simulink model "ECCE_demo1_model"  (R2020a)
settings: Solver=ode23t  StartTime=0.0  StopTime=10/60  MaxStep=50e-6  RelTol=1e-3  AbsTol=1e-3  EnableMultiTasking=on
libraries: powerlib x17
settings Model: Creator=Raymundo  LastModifiedBy=Renata
settings SolverCC: AutoScaleAbsTol=off  MaxConsecutiveMinStep=50  ZeroCrossAlgorithm=Adaptive
settings DataIOCC: ReturnWorkspaceOutputs=off
settings OptimizationCC: LifeSpan=inf
settings DebuggingCC: SFUnexpectedBacktrackingDiag=warning  SFNoUnconditionalDefaultTransitionDiag=warning  ArithmeticOperatorsInVariantConditions=warning
settings SFSimCC: SimUseLocalCustomCode=off  CustomCodeUndefinedFunction=UseInterfaceOnly
settings RTWCC: RTWUseLocalCustomCode=off
settings CodeAppCC: StateflowObjectComments=on
settings GRTTargetCC: TargetLangStandard=C89/C90 (ANSI)
settings ConfigComp: CovMetricSettings=dw  CovHtmlReporting=on  CovSaveCumulativeToWorkspaceVar=on  CovSaveSingleToWorkspaceVar=on  CovExternalEMLEnable=off
settings SimscapeCC: SimscapeNormalizeSystem=off

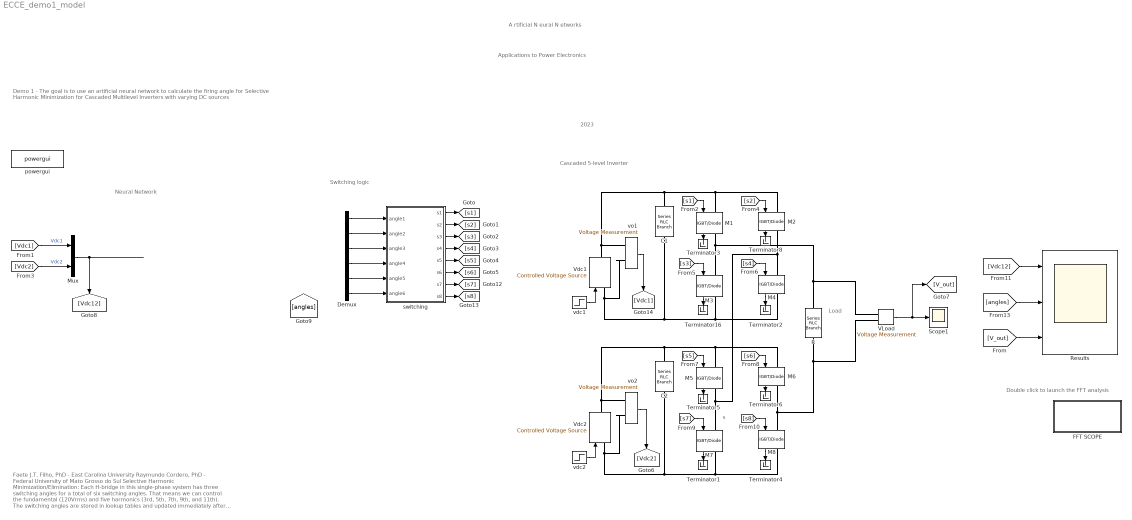
== system ECCE_demo1_model ==
  note: Double click to launch the FFT analysis
  note: Demo 1 - The goal is to use an artificial neural network to calculate the firing angle for Selective Harmonic Minimization for Cascaded Multilevel Inverters with varying DC sources
  note: Switching logic
  note: 2023
  note: A rtificial N eural N etworks
  note: Load
  note: Faete J.T. Filho, PhD - East Carolina University
      | Raymundo Cordero, PhD - Federal University of Mato Grosso do Sul
      |
      | Selective Harmonic Minimization/Elimination: Each H-bridge in this single-phase system has three switching angles for a total of six switching angles. That means we can control the fundamental (120Vrms) and five harmonics (3rd, 5th, 7th, 9th, and 11th). The switching angles are stored in lookup tables and updated immediately after the voltage changes, thus causing some harmonic distortion until a full cycle completes. The range of input voltage for which the harmonics are minimized/eliminated is from 110V to 140V.
      | Range of acceptable input voltage (Vdc1 & Vdc2) for SHE algorithm: 110V to 140V
  note: s
  note: Applications to Power Electronics
  note: Neural Network
  note: Cascaded 5-level Inverter
  C1 : powerlib/Elements/Series RLC Branch  LConnTagsString=__new0  RConnTagsString=__new0  BranchType=RC  Resistance=0.0001  Inductance=1e-3  SetiL0=off  InitialCurrent=0  Capacitance=5600e-6  Setx0=off  InitialVoltage=0  Measurements=None
  C2 : powerlib/Elements/Series RLC Branch  LConnTagsString=__new0  RConnTagsString=__new0  BranchType=RC  Resistance=0.0001  Inductance=1e-3  SetiL0=off  InitialCurrent=0  Capacitance=5600e-6  Setx0=off  InitialVoltage=0  Measurements=None
  Demux : Demux  Outputs=6
  FFT SCOPE : Subsystem
      settings: OpenFcn=power_fftscope
  M{1..8} (8 alike) : powerlib/Power Electronics/IGBT//Diode  Ron=1e-3  Rs=1e5  Cs=inf  Measurements=on
  Mux : Mux  Inputs=2
  R : powerlib/Elements/Series RLC Branch  LConnTagsString=__new0  RConnTagsString=__new0  BranchType=R  Resistance=100  Inductance=1e-3  SetiL0=off  InitialCurrent=0  Capacitance=5600e-6  Setx0=off  InitialVoltage=0  Measurements=None
  Results : Scope  NumInputPorts=3
  Scope1 : Scope
  Terminator{1..6,8,16} (8 alike) : Terminator
  VLoad : powerlib/Measurements/Voltage Measurement  PhasorSimulation=off  OutputType=Complex  PSBequivalent=0
  Vdc1 : powerlib/Electrical Sources/Controlled Voltage Source  Initialize=on  Source_Type=AC  Amplitude=0  Phase=0  Frequency=0  Measurements=None
  Vdc2 : powerlib/Electrical Sources/Controlled Voltage Source  Initialize=on  Source_Type=AC  Amplitude=0  Phase=0  Frequency=0  Measurements=None
  powergui : powerlib/powergui  Priority=1  SimulationMode=Continuous  SampleTime=50e-6  frequency=60  Iterations=50  frequencyindice=0  Pbase=100e6  ErrMax=1e-4  UnitsV=kV  UnitsW=MW  buscounter=0  FunctionMessages=off  echomessages=off  EnableUseOfTLC=off  CurrentSourceSwitches=off  DisableSnubberDevices=off  DisableRonSwitches=off  DisableVfSwitches=off  DisplayEquations=off  AutomaticDiscreteSolvers=off  SolverType=Tustin/Backward Euler (TBE)  Interpol=off  ExternalGateDelay=off  methode=off  Ts=100  x0status=blocks  SPID=on  SwTol=0  HookPort=off  NonlinearTolerance=1e-4  nMaxIteration=100  ContinueOnMaxIteration=off  RestoreLinks=warning  ResistiveCurrentMeasurement=off  Frange=[0:2:500]  Ylog=off  Xlog=on  ShowGrid=off  save=off  variable=ZData  structure=V_load  ZoomFFT=off  StartTime=0.1  cycles=3  DisplayStyle=1  fundamental=60  FreqAxis=on  MaxFrequency=2000  frequencyindicesteady=1  RmsSteady=1  display=off
  switching : Subsystem
  vdc1 : Step  Time=0.1  Before=115  After=130  SampleTime=0
  vdc2 : Step  Time=0.1  Before=125  After=135  SampleTime=0
  vo1 : powerlib/Measurements/Voltage Measurement  PhasorSimulation=off  OutputType=Complex  PSBequivalent=0
  vo2 : powerlib/Measurements/Voltage Measurement  PhasorSimulation=off  OutputType=Complex  PSBequivalent=0
  wires:
  M1/1 -> Terminator3/1
  M2/1 -> Terminator8/1
  [s1] -> M1/1
  [s2] -> M2/1
  [s3] -> M3/1
  [s4] -> M4/1
  [Vdc1] -> Mux/1  "Vdc1"
  [Vdc2] -> Mux/2  "Vdc2"
  vdc1/1 -> Vdc1/1
  Mux/1 -> [Vdc12]
  M4/1 -> Terminator2/1
  M3/1 -> Terminator16/1
  vo1/1 -> [Vdc1]
  M5/1 -> Terminator5/1
  M6/1 -> Terminator6/1
  [s5] -> M5/1
  [s6] -> M6/1
  [s7] -> M7/1
  [s8] -> M8/1
  vdc2/1 -> Vdc2/1
  M8/1 -> Terminator4/1
  M7/1 -> Terminator1/1
  vo2/1 -> [Vdc2]
  switching/1(s1) -> [s1]
  switching/2(s2) -> [s2]
  switching/3(s3) -> [s3]
  switching/4(s4) -> [s4]
  switching/5(s5) -> [s5]
  switching/6(s6) -> [s6]
  switching/7(s7) -> [s7]
  switching/8(s8) -> [s8]
  Demux/1 -> switching/1(angle1)
  Demux/2 -> switching/2(angle2)
  Demux/3 -> switching/3(angle3)
  Demux/4 -> switching/4(angle4)
  Demux/5 -> switching/5(angle5)
  Demux/6 -> switching/6(angle6)
  VLoad/1 -> Scope1/1, [V_out]
  ? -> Demux/1, [angles]  "Firing angle"
  [Vdc12] -> Results/1
  [V_out] -> Results/3
  [angles] -> Results/2
  connections:
  M2/LConn1 -- Vdc1/RConn1 -- vo1/LConn1 -- C1/LConn1 -- M1/LConn1
  C1/RConn1 -- Vdc1/LConn1 -- vo1/LConn2 -- M4/RConn1 -- M3/RConn1
  Vdc2/RConn1 -- vo2/LConn1 -- C2/LConn1 -- M5/LConn1 -- M6/LConn1
  Vdc2/LConn1 -- vo2/LConn2 -- C2/RConn1 -- M7/RConn1 -- M8/RConn1
  M1/RConn1 -- VLoad/LConn1 -- R/RConn1 -- M3/LConn1
  M7/LConn1 -- M4/LConn1 -- M2/RConn1 -- M5/RConn1
  M6/RConn1 -- R/LConn1 -- VLoad/LConn2 -- M8/LConn1

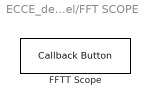
== system ECCE_demo1_model/FFT SCOPE ==
  FFTT Scope : CallbackButton  ButtonText=FFT analysis
      settings: ClickFcn=power_fftscope

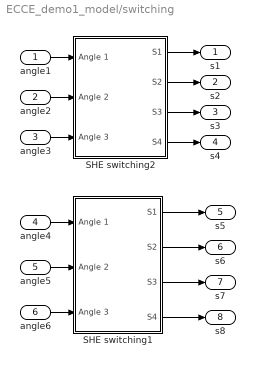
== system ECCE_demo1_model/switching ==
  angle1 : Inport
  angle2 : Inport  Port=2
  angle3 : Inport  Port=3
  angle4 : Inport  Port=4
  angle5 : Inport  Port=5
  angle6 : Inport  Port=6
  SHE switching1 : Subsystem
  SHE switching2 : Subsystem
  s1 : Outport
  s2 : Outport  Port=2
  s3 : Outport  Port=3
  s4 : Outport  Port=4
  s5 : Outport  Port=5
  s6 : Outport  Port=6
  s7 : Outport  Port=7
  s8 : Outport  Port=8
  wires:
  SHE switching2/1(S1) -> s1/1
  SHE switching1/1(S1) -> s5/1
  SHE switching2/4(S4) -> s4/1
  SHE switching1/4(S4) -> s8/1
  SHE switching2/2(S2) -> s2/1
  SHE switching2/3(S3) -> s3/1
  SHE switching1/3(S3) -> s7/1
  SHE switching1/2(S2) -> s6/1
  angle4/1 -> SHE switching1/1(Angle 1)
  angle6/1 -> SHE switching1/3(Angle 3)
  angle2/1 -> SHE switching2/2(Angle 2)
  angle5/1 -> SHE switching1/2(Angle 2)
  angle3/1 -> SHE switching2/3(Angle 3)
  angle1/1 -> SHE switching2/1(Angle 1)

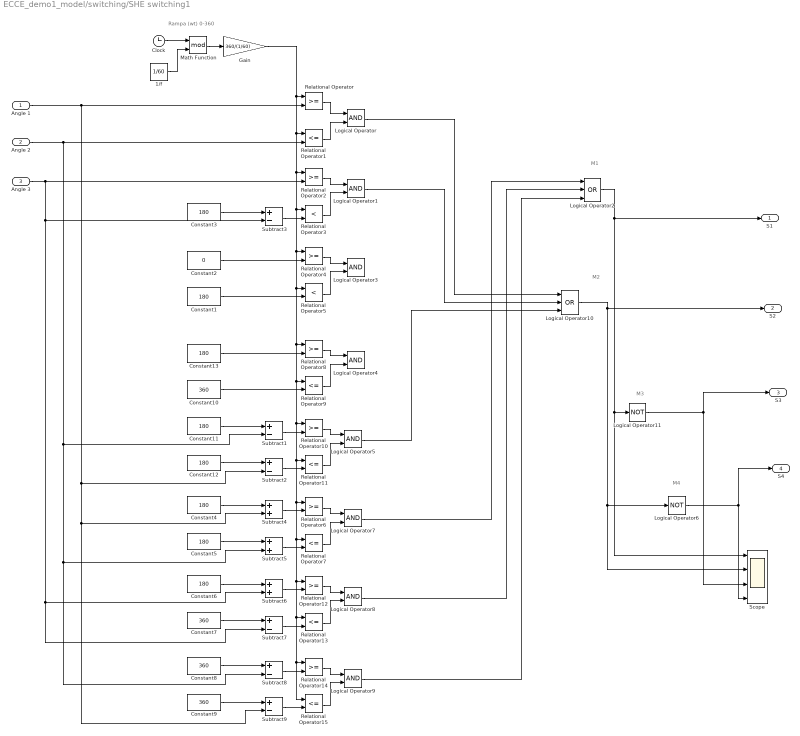
== system ECCE_demo1_model/switching/SHE switching1 ==
  note: M4
  note: M3
  note: M2
  note: M1
  note: Rampa (wt) 0-360
  Angle 1 : Inport
  Angle 2 : Inport  Port=2
  Angle 3 : Inport  Port=3
  1/f : Constant  Value=1/60
  Clock : Clock
  Constant{1,3..6,11..13} (8 alike) : Constant  Value=180
  Constant{7..10} (4 alike) : Constant  Value=360
  Constant2 : Constant  Value=0
  Gain : Gain  Gain=360/(1/60)
  Logical Operator{,1,3..5,7..9} (8 alike) : Logic  AllPortsSameDT=off  OutDataTypeStr=boolean
  Logical Operator10 : Logic  Operator=OR  Inputs=3  AllPortsSameDT=off  OutDataTypeStr=boolean
  Logical Operator11 : Logic  Operator=NOT  AllPortsSameDT=off  OutDataTypeStr=boolean
  Logical Operator2 : Logic  Operator=OR  Inputs=3  AllPortsSameDT=off  OutDataTypeStr=boolean
  Logical Operator6 : Logic  Operator=NOT  AllPortsSameDT=off  OutDataTypeStr=boolean
  Math Function : Math  Operator=mod  SignedPower=on  SaturateOnIntegerOverflow=on
  Relational Operator{,2,4,6,8,10,12,14} (8 alike) : RelationalOperator  OutDataTypeStr=boolean  RndMeth=Nearest
  Relational Operator{1,7,9,11,13,15} (6 alike) : RelationalOperator  Operator=<=  OutDataTypeStr=boolean  RndMeth=Nearest
  Relational Operator3 : RelationalOperator  Operator=<  OutDataTypeStr=boolean  RndMeth=Nearest
  Relational Operator5 : RelationalOperator  Operator=<  OutDataTypeStr=boolean  RndMeth=Nearest
  Scope : Scope  NumInputPorts=4
  Subtract{1..3,7..9} (6 alike) : Sum  Inputs=+-
  Subtract4 : Sum
  Subtract5 : Sum
  Subtract6 : Sum
  S1 : Outport
  S2 : Outport  Port=2
  S3 : Outport  Port=3
  S4 : Outport  Port=4
  wires:
  Gain/1 -> Relational Operator2/1, Relational Operator3/1, Relational Operator4/1, Relational Operator5/1, Relational Operator10/1, Relational Operator15/1, Relational Operator14/1, Relational Operator13/1, Relational Operator12/1, Relational Operator7/1, Relational Operator6/1, Relational Operator11/1, Relational Operator9/1, Relational Operator8/1, Relational Operator1/1, Relational Operator/1
  Relational Operator3/1 -> Logical Operator1/2
  Relational Operator10/1 -> Logical Operator5/1
  Relational Operator8/1 -> Logical Operator4/1
  1/f/1 -> Math Function/2
  Relational Operator1/1 -> Logical Operator/2
  Relational Operator2/1 -> Logical Operator1/1
  Relational Operator/1 -> Logical Operator/1
  Clock/1 -> Math Function/1
  Relational Operator11/1 -> Logical Operator5/2
  Relational Operator9/1 -> Logical Operator4/2
  Math Function/1 -> Gain/1
  Constant11/1 -> Subtract1/1
  Subtract1/1 -> Relational Operator10/2
  Subtract2/1 -> Relational Operator11/2
  Constant12/1 -> Subtract2/1
  Relational Operator4/1 -> Logical Operator3/1
  Relational Operator5/1 -> Logical Operator3/2
  Constant1/1 -> Relational Operator5/2
  Constant2/1 -> Relational Operator4/2
  Constant3/1 -> Subtract3/1
  Subtract3/1 -> Relational Operator3/2
  Constant5/1 -> Subtract5/1
  Subtract5/1 -> Relational Operator7/2
  Subtract4/1 -> Relational Operator6/2
  Constant4/1 -> Subtract4/1
  Relational Operator7/1 -> Logical Operator7/2
  Relational Operator6/1 -> Logical Operator7/1
  Relational Operator12/1 -> Logical Operator8/1
  Relational Operator13/1 -> Logical Operator8/2
  Constant6/1 -> Subtract6/1
  Subtract6/1 -> Relational Operator12/2
  Subtract7/1 -> Relational Operator13/2
  Angle 3/1 -> Relational Operator2/2, Subtract3/2, Subtract7/2, Subtract6/2
  Constant7/1 -> Subtract7/1
  Constant9/1 -> Subtract9/1
  Angle 1/1 -> Subtract9/2, Subtract4/2, Subtract2/2, Relational Operator/2
  Subtract9/1 -> Relational Operator15/2
  Subtract8/1 -> Relational Operator14/2
  Constant8/1 -> Subtract8/1
  Angle 2/1 -> Subtract8/2, Subtract5/2, Subtract1/2, Relational Operator1/2
  Relational Operator15/1 -> Logical Operator9/2
  Relational Operator14/1 -> Logical Operator9/1
  Logical Operator/1 -> Logical Operator10/1
  Logical Operator1/1 -> Logical Operator10/2
  Logical Operator5/1 -> Logical Operator10/3
  Logical Operator7/1 -> Logical Operator2/1
  Logical Operator8/1 -> Logical Operator2/2
  Logical Operator9/1 -> Logical Operator2/3
  Constant13/1 -> Relational Operator8/2
  Constant10/1 -> Relational Operator9/2
  Logical Operator2/1 -> Scope/1, Logical Operator11/1, S1/1
  Logical Operator10/1 -> Scope/2, Logical Operator6/1, S2/1
  Logical Operator11/1 -> S3/1, Scope/3
  Logical Operator6/1 -> Scope/4, S4/1

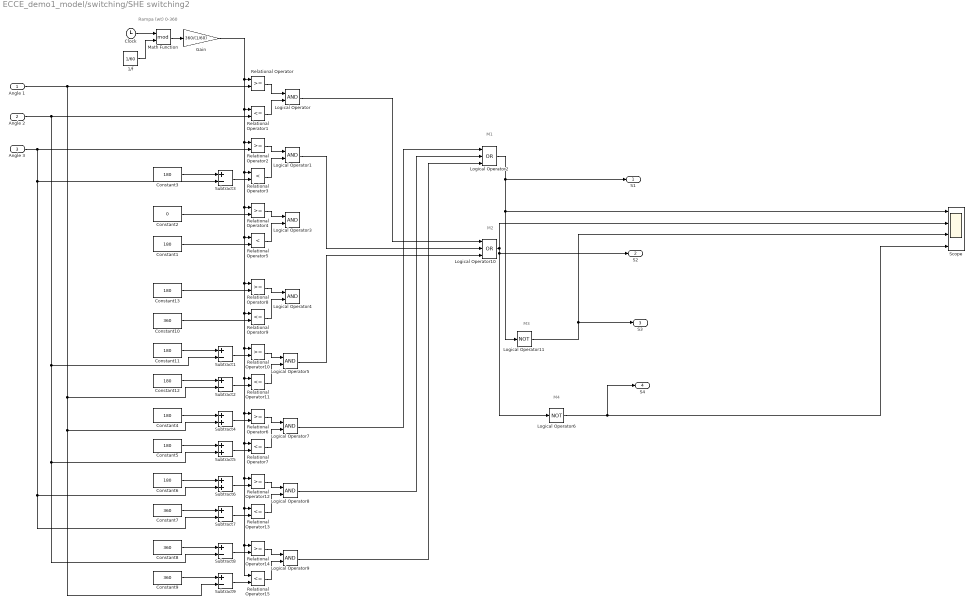
== system ECCE_demo1_model/switching/SHE switching2 ==
  note: M4
  note: M3
  note: M2
  note: M1
  note: Rampa (wt) 0-360
  Angle 1 : Inport
  Angle 2 : Inport  Port=2
  Angle 3 : Inport  Port=3
  1/f : Constant  Value=1/60
  Clock : Clock
  Constant{1,3..6,11..13} (8 alike) : Constant  Value=180
  Constant{7..10} (4 alike) : Constant  Value=360
  Constant2 : Constant  Value=0
  Gain : Gain  Gain=360/(1/60)
  Logical Operator{,1,3..5,7..9} (8 alike) : Logic  AllPortsSameDT=off  OutDataTypeStr=boolean
  Logical Operator10 : Logic  Operator=OR  Inputs=3  AllPortsSameDT=off  OutDataTypeStr=boolean
  Logical Operator11 : Logic  Operator=NOT  AllPortsSameDT=off  OutDataTypeStr=boolean
  Logical Operator2 : Logic  Operator=OR  Inputs=3  AllPortsSameDT=off  OutDataTypeStr=boolean
  Logical Operator6 : Logic  Operator=NOT  AllPortsSameDT=off  OutDataTypeStr=boolean
  Math Function : Math  Operator=mod  SignedPower=on  SaturateOnIntegerOverflow=on
  Relational Operator{,2,4,6,8,10,12,14} (8 alike) : RelationalOperator  OutDataTypeStr=boolean  RndMeth=Nearest
  Relational Operator{1,7,9,11,13,15} (6 alike) : RelationalOperator  Operator=<=  OutDataTypeStr=boolean  RndMeth=Nearest
  Relational Operator3 : RelationalOperator  Operator=<  OutDataTypeStr=boolean  RndMeth=Nearest
  Relational Operator5 : RelationalOperator  Operator=<  OutDataTypeStr=boolean  RndMeth=Nearest
  Scope : Scope  NumInputPorts=4
  Subtract{1..3,7..9} (6 alike) : Sum  Inputs=+-
  Subtract4 : Sum
  Subtract5 : Sum
  Subtract6 : Sum
  S1 : Outport
  S2 : Outport  Port=2
  S3 : Outport  Port=3
  S4 : Outport  Port=4
  wires:
  Gain/1 -> Relational Operator2/1, Relational Operator3/1, Relational Operator4/1, Relational Operator5/1, Relational Operator10/1, Relational Operator15/1, Relational Operator14/1, Relational Operator13/1, Relational Operator12/1, Relational Operator7/1, Relational Operator6/1, Relational Operator11/1, Relational Operator9/1, Relational Operator8/1, Relational Operator1/1, Relational Operator/1
  Relational Operator3/1 -> Logical Operator1/2
  Relational Operator10/1 -> Logical Operator5/1
  Relational Operator8/1 -> Logical Operator4/1
  1/f/1 -> Math Function/2
  Relational Operator1/1 -> Logical Operator/2
  Relational Operator2/1 -> Logical Operator1/1
  Relational Operator/1 -> Logical Operator/1
  Clock/1 -> Math Function/1
  Relational Operator11/1 -> Logical Operator5/2
  Relational Operator9/1 -> Logical Operator4/2
  Math Function/1 -> Gain/1
  Constant11/1 -> Subtract1/1
  Subtract1/1 -> Relational Operator10/2
  Subtract2/1 -> Relational Operator11/2
  Constant12/1 -> Subtract2/1
  Relational Operator4/1 -> Logical Operator3/1
  Relational Operator5/1 -> Logical Operator3/2
  Constant1/1 -> Relational Operator5/2
  Constant2/1 -> Relational Operator4/2
  Constant3/1 -> Subtract3/1
  Subtract3/1 -> Relational Operator3/2
  Constant5/1 -> Subtract5/1
  Subtract5/1 -> Relational Operator7/2
  Subtract4/1 -> Relational Operator6/2
  Constant4/1 -> Subtract4/1
  Relational Operator7/1 -> Logical Operator7/2
  Relational Operator6/1 -> Logical Operator7/1
  Relational Operator12/1 -> Logical Operator8/1
  Relational Operator13/1 -> Logical Operator8/2
  Constant6/1 -> Subtract6/1
  Subtract6/1 -> Relational Operator12/2
  Subtract7/1 -> Relational Operator13/2
  Angle 3/1 -> Relational Operator2/2, Subtract3/2, Subtract7/2, Subtract6/2
  Constant7/1 -> Subtract7/1
  Constant9/1 -> Subtract9/1
  Angle 1/1 -> Subtract9/2, Subtract4/2, Subtract2/2, Relational Operator/2
  Subtract9/1 -> Relational Operator15/2
  Subtract8/1 -> Relational Operator14/2
  Constant8/1 -> Subtract8/1
  Angle 2/1 -> Subtract8/2, Subtract5/2, Subtract1/2, Relational Operator1/2
  Relational Operator15/1 -> Logical Operator9/2
  Relational Operator14/1 -> Logical Operator9/1
  Logical Operator/1 -> Logical Operator10/1
  Logical Operator1/1 -> Logical Operator10/2
  Logical Operator5/1 -> Logical Operator10/3
  Logical Operator7/1 -> Logical Operator2/1
  Logical Operator8/1 -> Logical Operator2/2
  Logical Operator9/1 -> Logical Operator2/3
  Constant13/1 -> Relational Operator8/2
  Constant10/1 -> Relational Operator9/2
  Logical Operator2/1 -> Scope/1, Logical Operator11/1, S1/1
  Logical Operator10/1 -> Scope/2, S2/1, Logical Operator6/1
  Logical Operator11/1 -> Scope/3, S3/1
  Logical Operator6/1 -> Scope/4, S4/1
